simulink model "communicationHost"  (R2019a)
settings: Solver=FixedStepAuto  StartTime=0.0  StopTime=inf  FixedStep=Ts  RelTol=1e-3
undefined symbols (not defined in the file or in its folder): Ts
libraries: instrumentlib x5, dspsigops x3, aerolibanimutils x1, robotlib x1

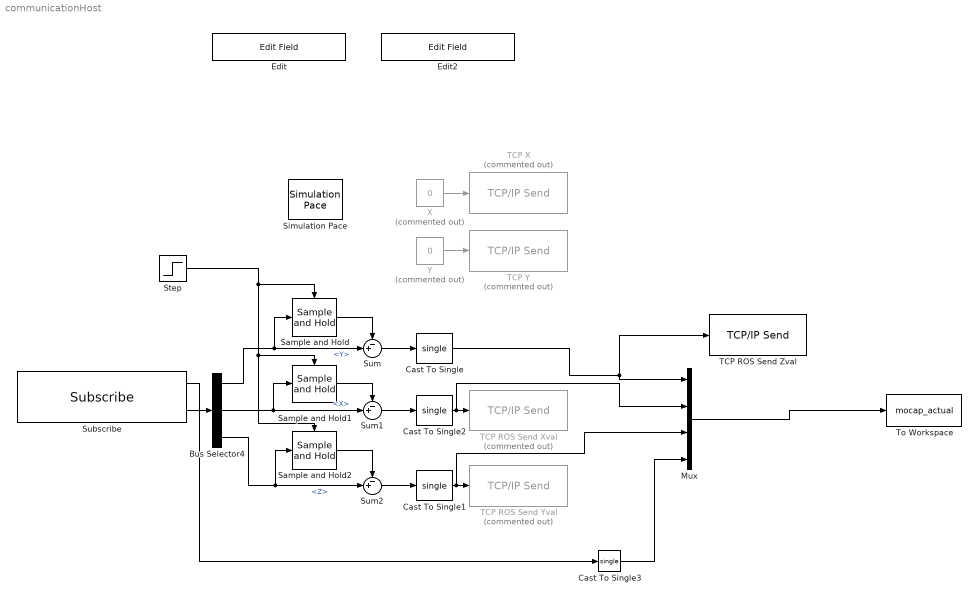
== system communicationHost ==
  Bus Selector4 : BusSelector  OutputSignals=Pose.Position.Y,Pose.Position.X,Pose.Position.Z
  Cast To Single{,1..3} (4 alike) : DataTypeConversion  OutDataTypeStr=single
  Edit : EditField  LabelPosition=Hide  ShowInitialText=on  Alignment=Center
  Edit2 : EditField  LabelPosition=Hide  ShowInitialText=on  Alignment=Center
  Mux : Mux
  Sample and Hold : dspsigops/Sample and Hold  trig=Rising edge  initCond=0  latchinput=off
  Sample and Hold1 : dspsigops/Sample and Hold  trig=Rising edge  initCond=0  latchinput=off
  Sample and Hold2 : dspsigops/Sample and Hold  trig=Rising edge  initCond=0  latchinput=off
  Simulation Pace : aerolibanimutils/Simulation Pace  SimulationPace=1  SleepMode=MATLAB Thread  OutputPaceError=off  SampleTime=Ts
  Step : Step  Time=Ts  SampleTime=0
  Subscribe : robotlib/Subscribe  topicSource=Select from ROS network  topic=/vrpn_client_node/robot1/pose  messageType=geometry_msgs/PoseStamped  sampleTime=Ts  messageQueueLength=1
  Sum : Sum  Inputs=-+|
  Sum1 : Sum  Inputs=-+|
  Sum2 : Sum  Inputs=-+|
  TCP ROS Send Xval : instrumentlib/TCP//IP Send  Commented=on  Host=192.168.3.1  Port=25001  EnableBlockingMode=off  Timeout=10  ByteOrder=BigEndian  TransferDelay=off
  TCP ROS Send Yval : instrumentlib/TCP//IP Send  Commented=on  Host=192.168.3.1  Port=25002  EnableBlockingMode=off  Timeout=10  ByteOrder=BigEndian  TransferDelay=off
  TCP ROS Send Zval : instrumentlib/TCP//IP Send  Host=192.168.3.1  Port=25000  EnableBlockingMode=off  Timeout=10  ByteOrder=BigEndian  TransferDelay=off
  TCP X : instrumentlib/TCP//IP Send  Commented=on  Host=192.168.3.1  Port=27001  EnableBlockingMode=off  Timeout=10  ByteOrder=BigEndian  TransferDelay=off
  TCP Y : instrumentlib/TCP//IP Send  Commented=on  Host=192.168.3.1  Port=27002  EnableBlockingMode=off  Timeout=10  ByteOrder=BigEndian  TransferDelay=off
  To Workspace : ToWorkspace  VariableName=mocap_actual  SaveFormat=Structure With Time  SampleTime=-1
  X : Constant  Commented=on  Value=0  OutDataTypeStr=single  SampleTime=Ts
  Y : Constant  Commented=on  Value=0  OutDataTypeStr=single  SampleTime=Ts
  wires:
  Subscribe/2 -> Bus Selector4/1
  Bus Selector4/1 -> Sample and Hold/1, Sum/2  "<Y>"
  Sum/1 -> Cast To Single/1
  Cast To Single/1 -> TCP ROS Send Zval/1, Mux/1
  X/1 -> TCP X/1
  Y/1 -> TCP Y/1
  Bus Selector4/3 -> Sample and Hold2/1, Sum2/2  "<Z>"
  Sum2/1 -> Cast To Single1/1
  Cast To Single1/1 -> Mux/3, TCP ROS Send Yval/1
  Sum1/1 -> Cast To Single2/1
  Cast To Single2/1 -> Mux/2, TCP ROS Send Xval/1
  Sample and Hold/1 -> Sum/1
  Bus Selector4/2 -> Sample and Hold1/1, Sum1/2  "<X>"
  Sample and Hold1/1 -> Sum1/1
  Sample and Hold2/1 -> Sum2/1
  Step/1 -> Sample and Hold2/Trigger, Sample and Hold1/Trigger, Sample and Hold/Trigger
  Subscribe/1 -> Cast To Single3/1
  Mux/1 -> To Workspace/1
  Cast To Single3/1 -> Mux/4
